simulink model "gm_sampleModel2011_sub_sub"  (R2023a)
settings: Solver=VariableStepAuto  StartTime=0.0  StopTime=10.0  RelTol=1e-3
libraries: hdlsllib x3, simulink x1
settings Model: Creator=user1  LastModifiedBy=user1
settings OptimizationCC: BlockReduction=off  ConditionallyExecuteInputs=off
settings DebuggingCC: InheritedTsInSrcMsg=none

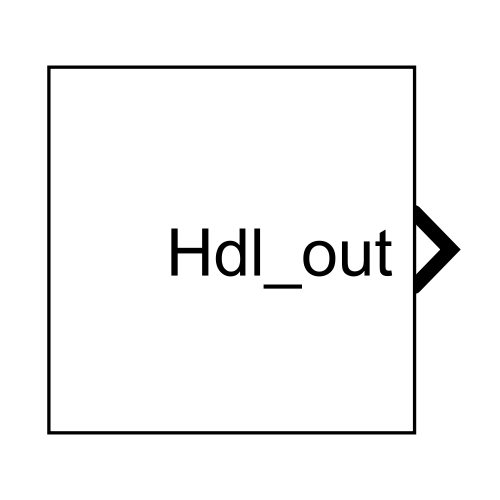
[thumbnail: Simulink's stored preview of the top-level diagram]
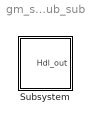
== system gm_sampleModel2011_sub_sub ==
  Subsystem : Subsystem

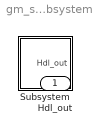
== system gm_sampleModel2011_sub_sub/Subsystem ==
  Subsystem : Subsystem
  Hdl_out : Outport  OutDataTypeStr=uint8

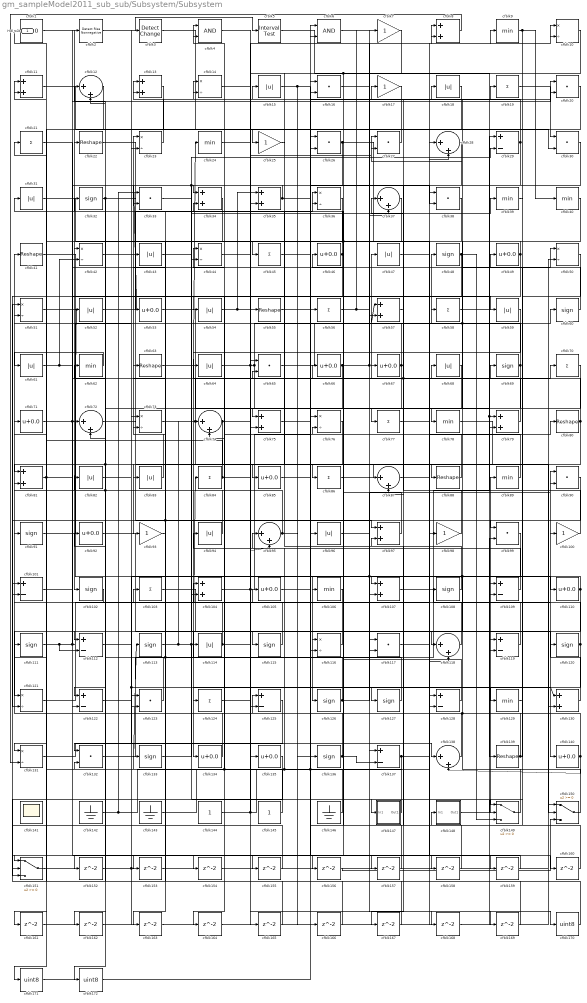
== system gm_sampleModel2011_sub_sub/Subsystem/Subsystem ==
  cfblk1 : hdlsllib/Logic and Bit Operations/Compare To Zero  relop=<=  OutDataTypeStr=uint8
  cfblk{10,14,23,36,42,44,50..51,73,76,116,121,131} (13 alike) : Product  Inputs=*/  OutDataTypeStr=uint8  RndMeth=Zero  SaturateOnIntegerOverflow=on
  cfblk{7,17,25,93,98,100} (6 alike) : Gain  OutDataTypeStr=uint8
  cfblk{29,101,109,112,119,122,125,128,137} (9 alike) : Sum  Inputs=+-  OutDataTypeStr=uint8
  cfblk{32,48,60,69,91,102,108,111,113,115,120,126..127,133,136} (15 alike) : Signum
  cfblk{19,21,45,56,58,70,77,84,86,103,124} (11 alike) : Sum  Inputs=+  OutDataTypeStr=uint8
  cfblk{8,11,13,34..35,57,75,79,81,97,104,107,130} (13 alike) : Sum  OutDataTypeStr=uint8
  cfblk{46,49,53,66..67,71,85,92,105,110,134..135,140} (13 alike) : Bias  Bias=0.0  SaturateOnIntegerOverflow=off
  cfblk{9,24,39..40,62,78,89,106,129} (9 alike) : MinMax  OutDataTypeStr=uint8
  cfblk{15,18,31,43,47,52,54,59,61,64,68,82..83,94,96,114} (16 alike) : Abs  OutDataTypeStr=uint8  SaturateOnIntegerOverflow=off
  cfblk{16,20,26..27,30,33,38,65,90,99,117,123,132} (13 alike) : DotProduct  OutDataTypeStr=uint8
  cfblk{12,28,37,72,74,87,95,118,138} (9 alike) : Sum  Inputs=|++  OutDataTypeStr=uint8
  cfblk{22,41,55,63,80,88,139} (7 alike) : Reshape
  cfblk141 : Scope
      settings: Floating=on
  cfblk142 : Ground
  cfblk143 : Ground
  cfblk144 : Constant  OutDataTypeStr=uint8  SampleTime=-1
  cfblk145 : Constant  OutDataTypeStr=uint8  SampleTime=-1
  cfblk146 : Ground
  cfblk147 : Subsystem
      settings: LibrarySourceBlock=|
      | hdlsllib/Ports &
      | Subsystems/Subsystem
  cfblk148 : Subsystem
      settings: LibrarySourceBlock=|
      | hdlsllib/Ports &
      | Subsystems/Subsystem
  cfblk149 : Switch  OutDataTypeStr=uint8  SaturateOnIntegerOverflow=off  InputSameDT=off
  cfblk150 : Switch  OutDataTypeStr=uint8  SaturateOnIntegerOverflow=off  InputSameDT=off
  cfblk151 : Switch  OutDataTypeStr=uint8  SaturateOnIntegerOverflow=off  InputSameDT=off
  cfblk{152..169} (18 alike) : Delay  SampleTime=1
  cfblk170 : DataTypeConversion  OutDataTypeStr=uint8  SaturateOnIntegerOverflow=off  RndMeth=Floor
  cfblk171 : DataTypeConversion  OutDataTypeStr=uint8  SaturateOnIntegerOverflow=off  RndMeth=Floor
  cfblk172 : DataTypeConversion  OutDataTypeStr=uint8  SaturateOnIntegerOverflow=off  RndMeth=Floor
  cfblk2 : hdlsllib/Logic and Bit Operations/Detect Rise Nonnegative  vinit=0  OutDataTypeStr=uint8
  cfblk3 : simulink/Logic and Bit Operations/Detect Change  vinit=0  OutDataTypeStr=uint8
      settings: LibrarySourceBlock=|
      | hdlsllib/Logic and Bit
      | Operations/Detect
      | Change
  cfblk4 : Logic  AllPortsSameDT=off  OutDataTypeStr=boolean
  cfblk5 : hdlsllib/Logic and Bit Operations/Interval Test  IntervalClosedRight=on  uplimit=0.5  IntervalClosedLeft=on  lowlimit=-0.5  OutDataTypeStr=uint8
  cfblk6 : Logic  AllPortsSameDT=off  OutDataTypeStr=boolean
  Hdl_out : Outport  OutDataTypeStr=uint8
  wires:
  cfblk54/1 -> cfblk59/1, cfblk35/1
  cfblk79/1 -> cfblk17/1, cfblk24/1
  cfblk136/1 -> cfblk137/2, cfblk41/1
  cfblk9/1 -> cfblk40/1, cfblk107/1
  cfblk52/1 -> cfblk36/1
  cfblk65/1 -> cfblk60/1
  cfblk27/1 -> cfblk102/1
  cfblk102/1 -> cfblk21/1
  cfblk10/1 -> cfblk75/1
  cfblk18/1 -> cfblk25/1
  cfblk2/1 -> cfblk5/1
  cfblk22/1 -> cfblk97/1
  cfblk107/1 -> cfblk90/1
  cfblk86/1 -> cfblk88/1
  cfblk1/1 -> cfblk22/1
  cfblk3/1 -> cfblk55/1
  cfblk12/1 -> cfblk151/1
  cfblk148/1(Out1) -> cfblk89/1
  cfblk143/1 -> cfblk16/1
  cfblk92/1 -> cfblk115/1
  cfblk104/1 -> cfblk8/2, cfblk16/2
  cfblk63/1 -> cfblk134/1
  cfblk83/1 -> cfblk23/1
  cfblk147/1(Out1) -> cfblk104/1, cfblk113/1
  cfblk51/1 -> cfblk126/1
  cfblk29/1 -> cfblk13/2, cfblk44/2, cfblk53/1
  cfblk4/1 -> cfblk107/2
  cfblk113/1 -> cfblk74/1, cfblk149/2, cfblk84/1
  cfblk132/1 -> cfblk29/1
  cfblk15/1 -> cfblk136/1, cfblk147/1(In1)
  cfblk47/1 -> cfblk108/1
  cfblk23/1 -> cfblk13/1
  cfblk138/1 -> cfblk125/1
  cfblk13/1 -> cfblk81/1
  cfblk114/1 -> cfblk169/1, cfblk91/1
  cfblk34/1 -> cfblk131/1
  cfblk127/1 -> cfblk114/1
  cfblk41/1 -> cfblk135/1
  cfblk48/1 -> cfblk149/3, cfblk127/1
  cfblk112/1 -> cfblk138/1
  cfblk94/1 -> cfblk32/1, cfblk52/1
  cfblk131/1 -> cfblk133/1
  cfblk25/1 -> cfblk85/1
  cfblk126/1 -> cfblk90/2, cfblk63/1, cfblk12/1
  cfblk130/1 -> cfblk100/1
  cfblk80/1 -> cfblk162/1, cfblk47/1
  cfblk8/1 -> cfblk131/2
  cfblk42/1 -> cfblk139/1
  cfblk76/1 -> cfblk93/1
  cfblk91/1 -> cfblk23/2
  cfblk124/1 -> cfblk69/1
  cfblk62/1 -> cfblk61/1
  cfblk99/1 -> cfblk118/1, cfblk123/2, cfblk117/2
  cfblk37/1 -> cfblk171/1, cfblk156/1
  cfblk111/1 -> cfblk112/2, cfblk20/2, cfblk103/1
  cfblk134/1 -> cfblk82/1
  cfblk145/1 -> cfblk44/1
  cfblk149/1 -> cfblk27/1, cfblk57/1
  cfblk73/1 -> cfblk117/1, cfblk67/1
  cfblk103/1 -> cfblk140/1
  cfblk123/1 -> cfblk62/1
  cfblk117/1 -> cfblk10/1
  cfblk28/1 -> cfblk42/1
  cfblk43/1 -> cfblk39/1
  cfblk105/1 -> cfblk26/1
  cfblk78/1 -> cfblk150/1
  cfblk100/1 -> cfblk15/1
  cfblk129/1 -> cfblk148/1(In1)
  cfblk58/1 -> cfblk119/1
  cfblk50/1 -> cfblk149/1
  cfblk36/1 -> cfblk83/1
  cfblk7/1 -> cfblk75/2, cfblk86/1
  cfblk20/1 -> cfblk116/1
  cfblk67/1 -> cfblk167/1, cfblk74/2, cfblk4/1
  cfblk115/1 -> cfblk4/2
  cfblk93/1 -> cfblk43/1
  cfblk35/1 -> cfblk38/2, cfblk34/1
  cfblk88/1 -> cfblk34/2
  cfblk106/1 -> cfblk121/1
  cfblk69/1 -> cfblk104/2, cfblk48/1
  cfblk72/1 -> cfblk150/2
  cfblk60/1 -> cfblk18/1
  cfblk140/1 -> cfblk14/1, cfblk138/2
  cfblk119/1 -> cfblk105/1
  cfblk5/1 -> cfblk79/1, cfblk109/1
  cfblk74/1 -> cfblk27/2, cfblk161/1, cfblk132/1
  cfblk128/1 -> cfblk76/2
  cfblk150/1 -> cfblk58/1
  cfblk40/1 -> cfblk78/1
  cfblk97/1 -> cfblk46/1
  cfblk137/1 -> cfblk132/2, cfblk118/2
  cfblk120/1 -> cfblk124/1, cfblk1/1
  cfblk109/1 -> cfblk94/1
  cfblk53/1 -> cfblk77/1
  cfblk70/1 -> cfblk116/2
  cfblk121/1 -> cfblk38/1
  cfblk59/1 -> cfblk64/1
  cfblk84/1 -> cfblk11/2, cfblk129/1
  cfblk82/1 -> cfblk70/1
  cfblk81/1 -> cfblk65/2, cfblk11/1
  cfblk95/1 -> cfblk166/1, cfblk81/2
  cfblk21/1 -> cfblk54/1
  cfblk133/1 -> cfblk29/2
  cfblk151/1 -> cfblk50/2, cfblk73/1
  cfblk33/1 -> cfblk120/1
  cfblk17/1 -> cfblk57/2
  cfblk146/1 -> cfblk95/1, cfblk14/2, cfblk111/1
  cfblk64/1 -> cfblk95/2, cfblk79/2, cfblk28/2
  cfblk110/1 -> cfblk154/1, cfblk106/1
  cfblk66/1 -> cfblk172/1, cfblk8/1, cfblk87/1
  cfblk26/1 -> cfblk122/2, cfblk128/2
  cfblk116/1 -> cfblk112/1
  cfblk87/1 -> cfblk80/1
  cfblk49/1 -> cfblk164/1, cfblk45/1
  cfblk16/1 -> cfblk137/1
  cfblk108/1 -> cfblk31/1
  cfblk135/1 -> cfblk151/3
  cfblk31/1 -> cfblk98/1
  cfblk61/1 -> cfblk42/2, cfblk2/1
  cfblk75/1 -> cfblk110/1
  cfblk89/1 -> cfblk51/2
  cfblk19/1 -> cfblk30/1
  cfblk45/1 -> cfblk20/1
  cfblk144/1 -> cfblk35/2, cfblk10/2, cfblk56/1
  cfblk98/1 -> cfblk37/1
  cfblk142/1 -> cfblk33/1, cfblk65/1
  cfblk11/1 -> cfblk37/2
  cfblk118/1 -> cfblk92/1
  cfblk32/1 -> cfblk96/1, cfblk122/1
  cfblk56/1 -> cfblk7/1, cfblk9/1
  cfblk85/1 -> cfblk19/1
  cfblk57/1 -> cfblk87/2
  cfblk38/1 -> cfblk125/2
  cfblk14/1 -> cfblk30/2
  cfblk39/1 -> cfblk99/1
  cfblk122/1 -> cfblk130/1, cfblk3/1
  cfblk46/1 -> cfblk12/2, cfblk101/2
  cfblk90/1 -> cfblk153/1, cfblk121/2
  cfblk139/1 -> cfblk49/1, cfblk68/1, cfblk66/1
  cfblk101/1 -> cfblk50/1, cfblk72/1
  cfblk125/1 -> cfblk152/1
  cfblk152/1 -> cfblk128/1
  cfblk153/1 -> cfblk99/2
  cfblk154/1 -> cfblk26/2
  cfblk71/1 -> cfblk155/1
  cfblk155/1 -> cfblk101/1
  cfblk156/1 -> cfblk150/3
  cfblk30/1 -> cfblk157/1
  cfblk157/1 -> cfblk36/2
  cfblk55/1 -> cfblk158/1
  cfblk158/1 -> cfblk97/2
  cfblk77/1 -> cfblk159/1
  cfblk159/1 -> cfblk151/2
  cfblk44/1 -> cfblk160/1
  cfblk160/1 -> cfblk76/1
  cfblk161/1 -> cfblk130/2
  cfblk162/1 -> cfblk123/1
  cfblk68/1 -> cfblk163/1
  cfblk163/1 -> cfblk28/1
  cfblk164/1 -> cfblk109/2
  cfblk24/1 -> cfblk165/1
  cfblk165/1 -> cfblk51/1
  cfblk166/1 -> cfblk73/2
  cfblk167/1 -> cfblk72/2
  cfblk96/1 -> cfblk168/1
  cfblk168/1 -> cfblk119/2
  cfblk169/1 -> cfblk33/2
  cfblk6/1 -> cfblk170/1
  cfblk170/1 -> cfblk71/1
  cfblk171/1 -> cfblk6/1
  cfblk172/1 -> cfblk6/2

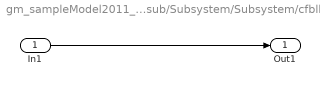
== system gm_sampleModel2011_sub_sub/Subsystem/Subsystem/cfblk147 ==
  In1 : Inport
  Out1 : Outport
  wires:
  In1/1 -> Out1/1

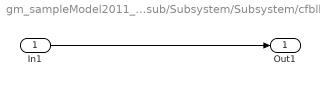
== system gm_sampleModel2011_sub_sub/Subsystem/Subsystem/cfblk148 ==
  In1 : Inport
  Out1 : Outport
  wires:
  In1/1 -> Out1/1
